simulink model "FastFourierTransform_Ex1"  (R2024a)
settings: Solver=ode45  StartTime=0.0  StopTime=4096  RelTol=1e-3  EnableMultiTasking=on
undefined symbols (not defined in the file): i, j, L, nsvg1369, xcvc1502
libraries: hdlBasic x15, aieUtilities x2, dspxfrm3 x1, hdlDSPIP x1, vmcUtilities x1
settings Model: Creator=dahlawat  LastModifiedBy=sdegala
settings SolverCC: AlgebraicLoopSolver=TrustRegion
settings DataIOCC: LimitDataPoints=on  SaveFormat=Array  ReturnWorkspaceOutputs=off
settings OptimizationCC: LifeSpan=inf
settings DebuggingCC: UnderspecifiedInitializationDetection=Classic  MergeDetectMultiDrivingBlocksExec=none  SolverPrmCheckMsg=warning  UnconnectedInputMsg=warning  UnconnectedOutputMsg=warning  UnconnectedLineMsg=warning  StateNameClashWarn=warning  SFUnexpectedBacktrackingDiag=warning  SFNoUnconditionalDefaultTransitionDiag=warning  SFExecutionAtInitializationDiag=none  ArithmeticOperatorsInVariantConditions=warning
settings HardwareCC: ProdBitPerPointer=32  ProdBitPerSizeT=32  ProdBitPerPtrDiffT=32  ProdLargestAtomicFloat=None  ProdIntDivRoundTo=Undefined  ProdEndianess=Unspecified  ProdWordSize=32  ProdHWDeviceType=32-bit Generic
settings ModelReferenceCC: EnableRefExpFcnMdlSchedulingChecks=on  PropagateSignalLabelsOutOfModel=off
settings SFSimCC: SimUseLocalCustomCode=off  CustomCodeUndefinedFunction=UseInterfaceOnly
settings RTWCC: RTWUseLocalCustomCode=off  GPUComputeCapability=3.5  DLArmComputeVersion=19.05
settings CodeAppCC: StateflowObjectComments=on
settings GRTTargetCC: TargetLangStandard=C89/C90 (ANSI)
settings ConfigComp: CovMetricSettings=dw  CovSaveCumulativeToWorkspaceVar=on  CovSaveSingleToWorkspaceVar=on  CovExternalEMLEnable=off

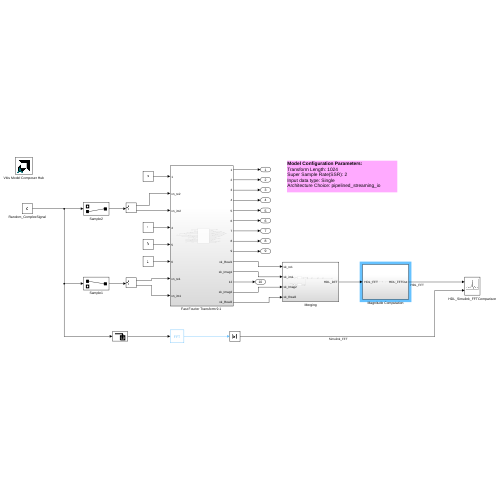
[thumbnail: Simulink's stored preview of the top-level diagram]
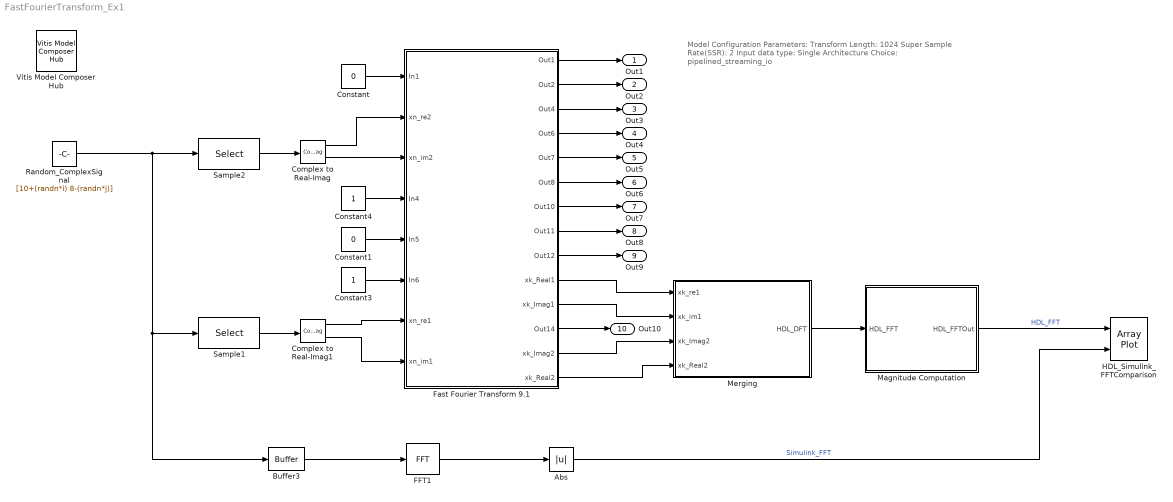
== system FastFourierTransform_Ex1 ==
  note: Model Configuration Parameters:
      | Transform Length: 1024
      | Super Sample Rate(SSR): 2
      | Input data type: Single
      | Architecture Choice: pipelined_streaming_io
  Abs : Abs  SaturateOnIntegerOverflow=off
  Buffer3 : Buffer  N=1024  OutputFrames=off
  Complex to Real-Imag : ComplexToRealImag
  Complex to Real-Imag1 : ComplexToRealImag
  Constant : Constant  Value=0  SampleTime=-1
  Constant1 : Constant  Value=0  SampleTime=-1
  Constant3 : Constant  OutDataTypeStr=single  SampleTime=-1
  Constant4 : Constant  SampleTime=-1
  FFT1 : dspxfrm3/FFT  FFTImplementation=FFTW  CompMethod=Table lookup  TableOpt=NEW  TableOptActive=Speed  BitRevOrder=on  Normalize=off  InheritFFTLength=on  FFTLength=64  WrapInput=on  roundingMode=Floor  overflowMode=off  firstCoeffDataTypeStr=Inherit: Same word length as input  firstCoeffLastDataTypeStr=Inherit: Same word length as input  outputMin=[]  outputMax=[]
  "Fast Fourier Transform 9.1 " : Subsystem
  HDL_Simulink_FFTComparison : ArrayPlot  NumInputPorts=2  WindowPosition=[1.000000,1.000000,1280.000000,744.000000,]  Visible=on  ScopeFrameLocation=window  YLimits=[474.75 477.25]  ShowLegend=on
  Magnitude Computation : Subsystem
  Merging : Subsystem
  Random_ComplexSignal : Constant  Value=[10+(randn*i) 8-(randn*j)]  OutDataTypeStr=single  SampleTime=1
  Sample1 : Selector  InputPortWidth=2  IndexOptions=Index vector (dialog)  Indices=1:2:2  OutputSizes=1
  Sample2 : Selector  InputPortWidth=2  IndexOptions=Index vector (dialog)  Indices=2:2:2  OutputSizes=1
  Vitis Model Composer Hub : vmcUtilities/Vitis Model Composer Hub  Tag=genX  CodeGeneration=off  SubsystemName=Fast Fourier Transform 9.1  StartColumn=1  NumberOfColumns=1  TargetDirectory=./code  exportDesign=off  analyzeDesign=off  validateDesignOnHw=off  ExportType=System Generator  IpVendor=xilinx.com  IpLibrary=hls  IpVersion=1.0  IpHWLanguage=Verilog  AieCompilerOptions={}  AieSimulatorOptions={}  CreateTestbench=off  TestbenchStackSize=10  RunRtlSim=off  RunCSim=off  RunAieSim=off  AieSimTimeout=50000  RunAieSimProfiling=off  LaunchVitisAnalyzer=off  PlotOutput=off  RunX86Sim=off  X86SimTimeout=10  GenHwImage=off  GenLibadfXo=on  GenHwValidationCode=off  PlatformType=Not Specified  HwSystemType=Baremetal  HwValidationTarget=hw  ProjDevice=xcvc1502-nsvg1369-1LHP-i-L  ProjDevicePart=xcvc1502-nsvg1369-1LHP-i-L  AIEType=AIE  SamplePeriod=-1  ClockFrequency=200  DataPathParallelism=1  xilinxfamily=versalaicore  part=xcvc1502  speed=-1LHP-i-L  package=nsvg1369  directory=./netlist/ip/Fast_Fourier_Transform_9.1_/src  testbench=off  incr_netlist=off  synthesis_tool=Vivado  clock_wrapper=Clock Enables  dbl_ovrd=According to Block Masks  dcm_input_clock_period=10  sysclk_period=4  simulink_period=1  eval_field=0  LogFileName=''  NThreads=4
  Out1 : Outport
  Out2 : Outport  Port=2
  Out3 : Outport  Port=3
  Out4 : Outport  Port=4
  Out5 : Outport  Port=5
  Out6 : Outport  Port=6
  Out7 : Outport  Port=7
  Out8 : Outport  Port=8
  Out9 : Outport  Port=9
  Out10 : Outport  Port=10
  wires:
  Constant/1 -> "Fast Fourier Transform 9.1 "/1(In1)
  Constant4/1 -> "Fast Fourier Transform 9.1 "/4(In4)
  Constant3/1 -> "Fast Fourier Transform 9.1 "/6(In6)
  Constant1/1 -> "Fast Fourier Transform 9.1 "/5(In5)
  Merging/1(HDL_DFT) -> Magnitude Computation/1(" HDL_FFT")
  Magnitude Computation/1(HDL_FFTOut) -> HDL_Simulink_FFTComparison/1  "HDL_FFT"
  "Fast Fourier Transform 9.1 "/10(xk_Real1) -> Merging/1(xk_re1)
  "Fast Fourier Transform 9.1 "/11(xk_Imag1) -> Merging/2(xk_im1)
  FFT1/1 -> Abs/1
  Abs/1 -> HDL_Simulink_FFTComparison/2  "Simulink_FFT"
  Buffer3/1 -> FFT1/1
  "Fast Fourier Transform 9.1 "/13(xk_Imag2) -> Merging/3(xk_Imag2)
  "Fast Fourier Transform 9.1 "/14(xk_Real2) -> Merging/4(xk_Real2)
  Sample2/1 -> Complex to Real-Imag/1
  Complex to Real-Imag/1 -> "Fast Fourier Transform 9.1 "/2(xn_re2)
  Complex to Real-Imag/2 -> "Fast Fourier Transform 9.1 "/3(xn_im2)
  Sample1/1 -> Complex to Real-Imag1/1
  Complex to Real-Imag1/1 -> "Fast Fourier Transform 9.1 "/7(xn_re1)
  Complex to Real-Imag1/2 -> "Fast Fourier Transform 9.1 "/8(xn_im1)
  Random_ComplexSignal/1 -> Buffer3/1, Sample1/1, Sample2/1
  "Fast Fourier Transform 9.1 "/1(Out1) -> Out1/1
  "Fast Fourier Transform 9.1 "/2(Out2) -> Out2/1
  "Fast Fourier Transform 9.1 "/3(Out4) -> Out3/1
  "Fast Fourier Transform 9.1 "/4(Out6) -> Out4/1
  "Fast Fourier Transform 9.1 "/5(Out7) -> Out5/1
  "Fast Fourier Transform 9.1 "/6(Out8) -> Out6/1
  "Fast Fourier Transform 9.1 "/7(Out10) -> Out7/1
  "Fast Fourier Transform 9.1 "/8(Out11) -> Out8/1
  "Fast Fourier Transform 9.1 "/9(Out12) -> Out9/1
  "Fast Fourier Transform 9.1 "/12(Out14) -> Out10/1

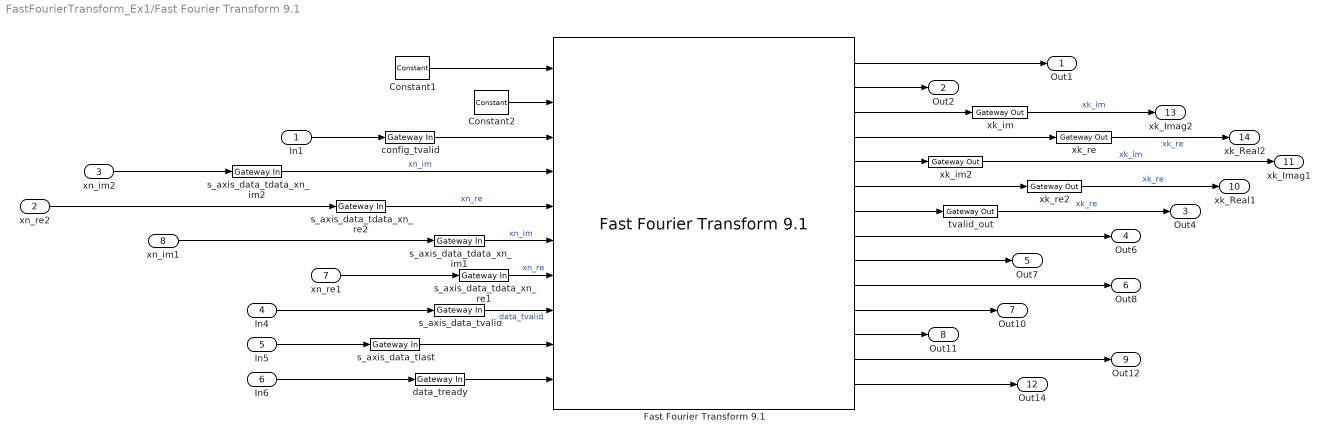
== system FastFourierTransform_Ex1/Fast Fourier Transform 9.1  ==
  In1 : Inport
  xn_re2 : Inport  Port=2
  xn_im2 : Inport  Port=3
  In4 : Inport  Port=4
  In5 : Inport  Port=5
  In6 : Inport  Port=6
  xn_re1 : Inport  Port=7
  xn_im1 : Inport  Port=8
  Constant1 : hdlBasic/Constant  const=683  gui_display_data_type=Fixed-point  arith_type=Unsigned  n_bits=10  bin_pt=0  preci_type=Single  exp_width=8  frac_width=24  explicit_period=on  period=1  XmcBlockStatus=1  maskContainerNames=tabcontainer1  block_type=constant  block_config=sysgen:Constant_config
  Constant2 : hdlBasic/Constant  const=1  gui_display_data_type=Fixed-point  arith_type=Unsigned  n_bits=1  bin_pt=0  preci_type=Single  exp_width=8  frac_width=24  explicit_period=on  period=1  XmcBlockStatus=1  maskContainerNames=tabcontainer1  block_type=constant  block_config=sysgen:Constant_config
  "Fast Fourier Transform 9.1 " : hdlDSPIP/Fast Fourier Transform 9.1   transform_length=1024  target_clock_frequency=250  target_data_throughput=50  implementation_options=pipelined_streaming_io  run_time_configurable_transform_length=off  enable_ssr=on  super_sample_rates=2  data_format=native_floating_point  phase_factor_width=24  scaling_options=scaled  rounding_modes=truncation  aclken=off  aresetn=off  output_ordering=natural_order  cyclic_prefix_insertion=off  throttle_scheme=nonrealtime  xk_index=off  ovflo=off  trim_axipin_name=on  memory_options_data=block_ram  memory_options_phase_factors=block_ram  number_of_stages_using_block_ram_for_data_and_phase_factors=1  memory_options_reorder=block_ram  memory_options_hybrid=off  complex_mult_type=use_mults_resources  butterfly_type=use_luts  simulation_type=hybrid_sim  simulation_model=sysgen:xfftv9_cmodel  data_path_portlist={ 's_axis_data_tdata', 'm_axis_data_tdata', 'm_axis_status_tdata', 'event_fft_overflow' }  channels=1  input_ordering=natural_order  input_width=16  ip_name=Fast Fourier Transform  ip_version=9.1  dsptool_ready=true  ipcore_usecache=true  ipcore_useipmodelcache=true  wrapper_available=true  port_translation_map={ 'aclken' => 'en', 'aresetn' => 'rst'}  XmcBlockStatus=1  maskContainerNames=tabcontainer1  block_type=xfft_v9_1  block_config=sysgen:rodinimport_config
  config_tvalid : hdlBasic/Gateway In  gui_display_data_type=Boolean  arith_type=Boolean  n_bits=16  bin_pt=15  preci_type=Single  exp_width=8  frac_width=24  rows=1  columns=1  quantization="Round  (unbiased: +/- Inf)"  overflow=Saturate  period=1  UseAsADC=off  ADCChannel='1'  interface=None  automatic_assignment=on  address_offset=hex2dec('00')  intf_name=''  intf_description=''  default_value=0  timing_constraint=None  locs_specified=off  LOCs={}  io_standard={}  inherit_from_input=off  hdl_port=on  XmcBlockStatus=1  maskContainerNames=group4  block_type=gatewayin  block_config=sysgen:gateway_in_config  block_width_w=590  block_height_w=620  block_width=640  block_height=850
  data_tready : hdlBasic/Gateway In  gui_display_data_type=Boolean  arith_type=Boolean  n_bits=16  bin_pt=15  preci_type=Single  exp_width=8  frac_width=24  rows=1  columns=1  quantization="Round  (unbiased: +/- Inf)"  overflow=Saturate  period=1  UseAsADC=off  ADCChannel='1'  interface=None  automatic_assignment=on  address_offset=hex2dec('00')  intf_name=''  intf_description=''  default_value=0  timing_constraint=None  locs_specified=off  LOCs={}  io_standard={}  inherit_from_input=off  hdl_port=on  XmcBlockStatus=1  maskContainerNames=group4  block_type=gatewayin  block_config=sysgen:gateway_in_config  block_width_w=590  block_height_w=620  block_width=640  block_height=850
  s_axis_data_tdata_xn_im1 : hdlBasic/Gateway In  gui_display_data_type=Floating-point  arith_type=Floating-point  n_bits=16  bin_pt=15  preci_type=Single  exp_width=8  frac_width=24  rows=1  columns=1  quantization="Round  (unbiased: +/- Inf)"  overflow=Saturate  period=1  UseAsADC=off  ADCChannel='1'  interface=None  automatic_assignment=on  address_offset=hex2dec('00')  intf_name=''  intf_description=''  default_value=0  timing_constraint=None  locs_specified=off  LOCs={}  io_standard={}  inherit_from_input=off  hdl_port=on  XmcBlockStatus=1  maskContainerNames=group4  block_type=gatewayin  block_config=sysgen:gateway_in_config  block_width_w=590  block_height_w=620  block_width=640  block_height=850
  s_axis_data_tdata_xn_im2 : hdlBasic/Gateway In  gui_display_data_type=Floating-point  arith_type=Floating-point  n_bits=16  bin_pt=15  preci_type=Single  exp_width=8  frac_width=24  rows=1  columns=1  quantization="Round  (unbiased: +/- Inf)"  overflow=Saturate  period=1  UseAsADC=off  ADCChannel='1'  interface=None  automatic_assignment=on  address_offset=hex2dec('00')  intf_name=''  intf_description=''  default_value=0  timing_constraint=None  locs_specified=off  LOCs={}  io_standard={}  inherit_from_input=off  hdl_port=on  XmcBlockStatus=1  maskContainerNames=group4  block_type=gatewayin  block_config=sysgen:gateway_in_config  block_width_w=590  block_height_w=620  block_width=640  block_height=850
  s_axis_data_tdata_xn_re1 : hdlBasic/Gateway In  gui_display_data_type=Floating-point  arith_type=Floating-point  n_bits=16  bin_pt=15  preci_type=Single  exp_width=8  frac_width=24  rows=1  columns=1  quantization="Round  (unbiased: +/- Inf)"  overflow=Saturate  period=1  UseAsADC=off  ADCChannel='1'  interface=None  automatic_assignment=on  address_offset=hex2dec('00')  intf_name=''  intf_description=''  default_value=0  timing_constraint=None  locs_specified=off  LOCs={}  io_standard={}  inherit_from_input=off  hdl_port=on  XmcBlockStatus=1  maskContainerNames=group4  block_type=gatewayin  block_config=sysgen:gateway_in_config  block_width_w=590  block_height_w=620  block_width=640  block_height=850
  s_axis_data_tdata_xn_re2 : hdlBasic/Gateway In  gui_display_data_type=Floating-point  arith_type=Floating-point  n_bits=16  bin_pt=15  preci_type=Single  exp_width=8  frac_width=24  rows=1  columns=1  quantization="Round  (unbiased: +/- Inf)"  overflow=Saturate  period=1  UseAsADC=off  ADCChannel='1'  interface=None  automatic_assignment=on  address_offset=hex2dec('00')  intf_name=''  intf_description=''  default_value=0  timing_constraint=None  locs_specified=off  LOCs={}  io_standard={}  inherit_from_input=off  hdl_port=on  XmcBlockStatus=1  maskContainerNames=group4  block_type=gatewayin  block_config=sysgen:gateway_in_config  block_width_w=590  block_height_w=620  block_width=640  block_height=850
  s_axis_data_tlast : hdlBasic/Gateway In  gui_display_data_type=Boolean  arith_type=Boolean  n_bits=9  bin_pt=8  preci_type=Single  exp_width=8  frac_width=24  rows=1  columns=1  quantization="Round  (unbiased: +/- Inf)"  overflow=Saturate  period=1  UseAsADC=off  ADCChannel='1'  interface=None  automatic_assignment=on  address_offset=hex2dec('00')  intf_name=''  intf_description=''  default_value=0  timing_constraint=None  locs_specified=off  LOCs={}  io_standard={}  inherit_from_input=off  hdl_port=on  XmcBlockStatus=1  maskContainerNames=group4  block_type=gatewayin  block_config=sysgen:gateway_in_config  block_width_w=590  block_height_w=620  block_width=640  block_height=850
  s_axis_data_tvalid : hdlBasic/Gateway In  gui_display_data_type=Boolean  arith_type=Boolean  n_bits=9  bin_pt=8  preci_type=Single  exp_width=8  frac_width=24  rows=1  columns=1  quantization="Round  (unbiased: +/- Inf)"  overflow=Saturate  period=1  UseAsADC=off  ADCChannel='1'  interface=None  automatic_assignment=on  address_offset=hex2dec('00')  intf_name=''  intf_description=''  default_value=0  timing_constraint=None  locs_specified=off  LOCs={}  io_standard={}  inherit_from_input=off  hdl_port=on  XmcBlockStatus=1  maskContainerNames=group4  block_type=gatewayin  block_config=sysgen:gateway_in_config  block_width_w=590  block_height_w=620  block_width=640  block_height=850
  tvalid_out : hdlBasic/Gateway Out  inherit_from_input=off  hdl_port=on  rows=1  columns=1  UseAsDAC=off  DACChannel='1'  interface=None  automatic_assignment=on  address_offset=hex2dec('00')  intf_name=''  intf_description=''  timing_constraint=None  locs_specified=off  LOCs={}  io_standard={}  XmcBlockStatus=1  maskContainerNames=group4  block_type=gatewayout  block_config=sysgen:gateway_out_config  block_width_w=590  block_height_w=620  block_width=620  block_height=750
  xk_im : hdlBasic/Gateway Out  inherit_from_input=off  hdl_port=on  rows=1  columns=1  UseAsDAC=off  DACChannel='1'  interface=None  automatic_assignment=on  address_offset=hex2dec('00')  intf_name=''  intf_description=''  timing_constraint=None  locs_specified=off  LOCs={}  io_standard={}  XmcBlockStatus=1  maskContainerNames=group4  block_type=gatewayout  block_config=sysgen:gateway_out_config  block_width_w=590  block_height_w=620  block_width=620  block_height=750
  xk_im2 : hdlBasic/Gateway Out  inherit_from_input=off  hdl_port=on  rows=1  columns=1  UseAsDAC=off  DACChannel='1'  interface=None  automatic_assignment=on  address_offset=hex2dec('00')  intf_name=''  intf_description=''  timing_constraint=None  locs_specified=off  LOCs={}  io_standard={}  XmcBlockStatus=1  maskContainerNames=group4  block_type=gatewayout  block_config=sysgen:gateway_out_config  block_width_w=590  block_height_w=620  block_width=620  block_height=750
  xk_re : hdlBasic/Gateway Out  inherit_from_input=off  hdl_port=on  rows=1  columns=1  UseAsDAC=off  DACChannel='1'  interface=None  automatic_assignment=on  address_offset=hex2dec('00')  intf_name=''  intf_description=''  timing_constraint=None  locs_specified=off  LOCs={}  io_standard={}  XmcBlockStatus=1  maskContainerNames=group4  block_type=gatewayout  block_config=sysgen:gateway_out_config  block_width_w=590  block_height_w=620  block_width=620  block_height=750
  xk_re2 : hdlBasic/Gateway Out  inherit_from_input=off  hdl_port=on  rows=1  columns=1  UseAsDAC=off  DACChannel='1'  interface=None  automatic_assignment=on  address_offset=hex2dec('00')  intf_name=''  intf_description=''  timing_constraint=None  locs_specified=off  LOCs={}  io_standard={}  XmcBlockStatus=1  maskContainerNames=group4  block_type=gatewayout  block_config=sysgen:gateway_out_config  block_width_w=590  block_height_w=620  block_width=620  block_height=750
  Out1 : Outport
  Out2 : Outport  Port=2
  Out4 : Outport  Port=3
  Out6 : Outport  Port=4
  Out7 : Outport  Port=5
  Out8 : Outport  Port=6
  Out10 : Outport  Port=7
  Out11 : Outport  Port=8
  Out12 : Outport  Port=9
  xk_Real1 : Outport  Port=10
  xk_Imag1 : Outport  Port=11
  Out14 : Outport  Port=12
  xk_Imag2 : Outport  Port=13
  xk_Real2 : Outport  Port=14
  wires:
  config_tvalid/1 -> "Fast Fourier Transform 9.1 "/3
  xk_re/1 -> xk_Real2/1  "xk_re"
  s_axis_data_tdata_xn_re2/1 -> "Fast Fourier Transform 9.1 "/5  "xn_re"
  In6/1 -> data_tready/1
  xk_im/1 -> xk_Imag2/1  "xk_im"
  In4/1 -> s_axis_data_tvalid/1
  s_axis_data_tdata_xn_im2/1 -> "Fast Fourier Transform 9.1 "/4  "xn_im"
  In1/1 -> config_tvalid/1
  "Fast Fourier Transform 9.1 "/2 -> Out2/1
  Constant2/1 -> "Fast Fourier Transform 9.1 "/2
  "Fast Fourier Transform 9.1 "/1 -> Out1/1
  xn_re2/1 -> s_axis_data_tdata_xn_re2/1
  xn_im2/1 -> s_axis_data_tdata_xn_im2/1
  "Fast Fourier Transform 9.1 "/13 -> Out12/1
  In5/1 -> s_axis_data_tlast/1
  xk_im2/1 -> xk_Imag1/1  "xk_im"
  xk_re2/1 -> xk_Real1/1  "xk_re"
  xn_re1/1 -> s_axis_data_tdata_xn_re1/1
  xn_im1/1 -> s_axis_data_tdata_xn_im1/1
  s_axis_data_tvalid/1 -> "Fast Fourier Transform 9.1 "/8  "data_tvalid"
  "Fast Fourier Transform 9.1 "/5 -> xk_im2/1
  "Fast Fourier Transform 9.1 "/6 -> xk_re2/1
  "Fast Fourier Transform 9.1 "/8 -> Out6/1
  "Fast Fourier Transform 9.1 "/9 -> Out7/1
  "Fast Fourier Transform 9.1 "/10 -> Out8/1
  "Fast Fourier Transform 9.1 "/11 -> Out10/1
  "Fast Fourier Transform 9.1 "/12 -> Out11/1
  Constant1/1 -> "Fast Fourier Transform 9.1 "/1
  s_axis_data_tdata_xn_im1/1 -> "Fast Fourier Transform 9.1 "/6  "xn_im"
  s_axis_data_tdata_xn_re1/1 -> "Fast Fourier Transform 9.1 "/7  "xn_re"
  "Fast Fourier Transform 9.1 "/3 -> xk_im/1
  "Fast Fourier Transform 9.1 "/4 -> xk_re/1
  s_axis_data_tlast/1 -> "Fast Fourier Transform 9.1 "/9
  data_tready/1 -> "Fast Fourier Transform 9.1 "/10
  "Fast Fourier Transform 9.1 "/14 -> Out14/1
  "Fast Fourier Transform 9.1 "/7 -> tvalid_out/1
  tvalid_out/1 -> Out4/1  "xk_re"

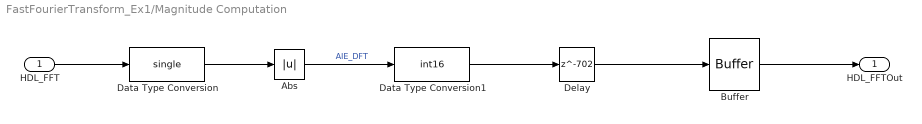
== system FastFourierTransform_Ex1/Magnitude Computation ==
  " HDL_FFT" : Inport
  Abs : Abs  SaturateOnIntegerOverflow=off
  Buffer : Buffer  N=1024  OutputFrames=off
  Data Type Conversion : DataTypeConversion  OutDataTypeStr=single  SaturateOnIntegerOverflow=off  RndMeth=Floor
  Data Type Conversion1 : DataTypeConversion  OutDataTypeStr=int16  SaturateOnIntegerOverflow=off  RndMeth=Floor
  Delay : Delay  DelayLength=702  InitialCondition=0
  HDL_FFTOut : Outport
  wires:
  Data Type Conversion/1 -> Abs/1
  Abs/1 -> Data Type Conversion1/1  "AIE_DFT"
  " HDL_FFT"/1 -> Data Type Conversion/1
  Data Type Conversion1/1 -> Delay/1
  Buffer/1 -> HDL_FFTOut/1
  Delay/1 -> Buffer/1

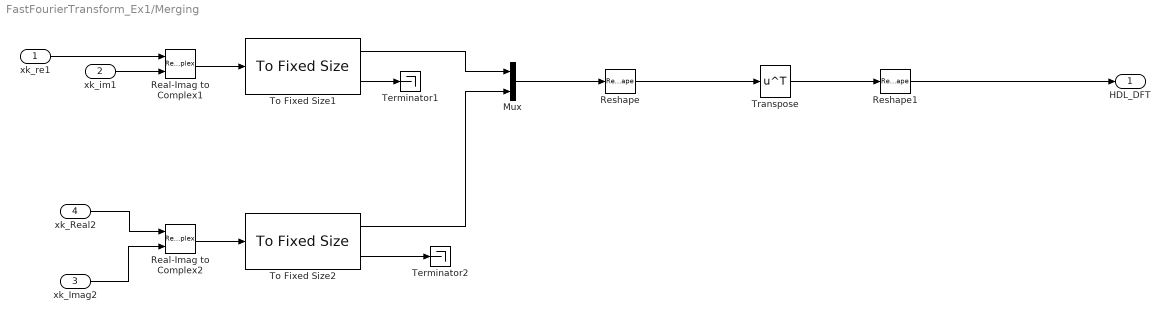
== system FastFourierTransform_Ex1/Merging ==
  xk_re1 : Inport
  xk_im1 : Inport  Port=2
  xk_Imag2 : Inport  Port=3
  xk_Real2 : Inport  Port=4
  Mux : Mux  Inputs=2
  Real-Imag to Complex1 : RealImagToComplex
  Real-Imag to Complex2 : RealImagToComplex
  Reshape : Reshape  OutputDimensionality=Customize  OutputDimensions=[1, 2]
  Reshape1 : Reshape  OutputDimensions=[1, 10]
  Terminator1 : Terminator
  Terminator2 : Terminator
  To Fixed Size1 : aieUtilities/To Fixed Size  Mode=Produce a valid output signal  OutputSize=Inherit: Same as input  CopyMethod=Buffer samples to form output  HasStatusOutput=on
  To Fixed Size2 : aieUtilities/To Fixed Size  Mode=Produce a valid output signal  OutputSize=Inherit: Same as input  CopyMethod=Buffer samples to form output  HasStatusOutput=on
  Transpose : Math  Operator=transpose
  HDL_DFT : Outport
  wires:
  xk_re1/1 -> Real-Imag to Complex1/1
  xk_im1/1 -> Real-Imag to Complex1/2
  To Fixed Size1/2 -> Terminator1/1
  Real-Imag to Complex1/1 -> To Fixed Size1/1
  xk_Real2/1 -> Real-Imag to Complex2/1
  xk_Imag2/1 -> Real-Imag to Complex2/2
  Real-Imag to Complex2/1 -> To Fixed Size2/1
  To Fixed Size2/2 -> Terminator2/1
  To Fixed Size1/1 -> Mux/1
  To Fixed Size2/1 -> Mux/2
  Reshape/1 -> Transpose/1
  Mux/1 -> Reshape/1
  Transpose/1 -> Reshape1/1
  Reshape1/1 -> HDL_DFT/1
